simulink model "Linear_System"  (R2020a)
settings: Solver=ode4  StartTime=0.0  StopTime=10.0  RelTol=1e-3
values from neighbouring files (symbols this model uses):
  A = [0 0 0 1 0 0 ... (first row only)    [Aircraft_parameters.m]
  B = [0 0 ... (first row only)    [Aircraft_parameters.m]
  C = eye(3,6)    [Aircraft_parameters.m]
  L = place(A', C', pl)'    [main.m]
  use_output = 0    [main.m]
  use_state = 1    [main.m]
  x_bar = [0 0 0 0 0 0]'    [Aircraft_parameters.m]
  x_inital = x0-x_bar    [Aircraft_parameters.m]
undefined symbols (not defined in the file or in its folder): K
settings Model: Creator=james  LastModifiedBy=connor

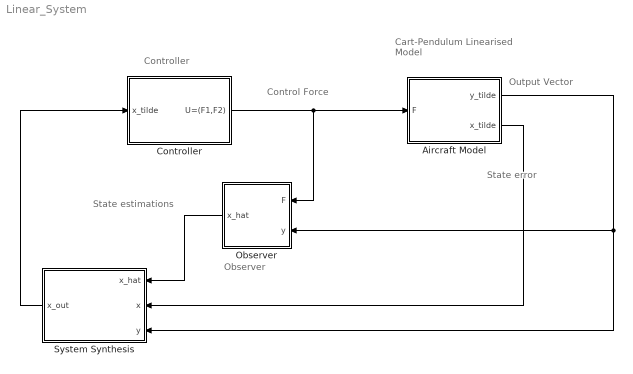
== system Linear_System ==
  note: Control Force
  note: Controller
  note: Cart-Pendulum
      | Linearised Model
  note: Output Vector
  note: Observer
  note: State error
  note: State estimations
  "Aircraft Model " : Subsystem
  Controller : Subsystem
  Observer : Subsystem
  System Synthesis : Subsystem
  wires:
  Controller/1(U=(F1,F2)) -> Observer/1(F), "Aircraft Model "/1(F)
  "Aircraft Model "/1(y_tilde) -> System Synthesis/3(y), Observer/2(y)
  "Aircraft Model "/2(x_tilde) -> System Synthesis/2(x)
  Observer/1(x_hat) -> System Synthesis/1(x_hat)
  System Synthesis/1(x_out) -> Controller/1(x_tilde)

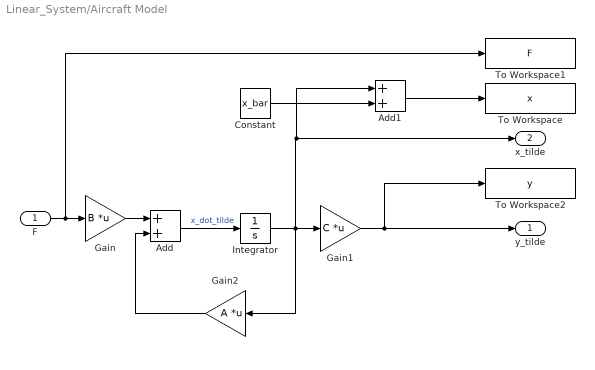
== system Linear_System/Aircraft Model  ==
  F : Inport
  Add : Sum
  Add1 : Sum
  Constant : Constant  Value=x_bar
  Gain : Gain  Gain=B  Multiplication=Matrix(K*u)
  Gain1 : Gain  Gain=C  Multiplication=Matrix(K*u)
  Gain2 : Gain  Gain=A  Multiplication=Matrix(K*u)
  Integrator : Integrator  InitialCondition=x_inital
  To Workspace : ToWorkspace  VariableName=x  SampleTime=-1
  To Workspace1 : ToWorkspace  VariableName=F  SampleTime=-1
  To Workspace2 : ToWorkspace  VariableName=y  SampleTime=-1
  y_tilde : Outport
  x_tilde : Outport  Port=2
  wires:
  F/1 -> Gain/1, To Workspace1/1
  Gain/1 -> Add/1
  Add/1 -> Integrator/1  "x_dot_tilde"
  Gain2/1 -> Add/2
  Integrator/1 -> Gain2/1, Add1/1, x_tilde/1, Gain1/1
  Gain1/1 -> y_tilde/1, To Workspace2/1
  Add1/1 -> To Workspace/1
  Constant/1 -> Add1/2

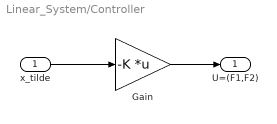
== system Linear_System/Controller ==
  x_tilde : Inport
  Gain : Gain  Gain=-K  Multiplication=Matrix(K*u)
  U=(F1,F2) : Outport
  wires:
  x_tilde/1 -> Gain/1
  Gain/1 -> U=(F1,F2)/1

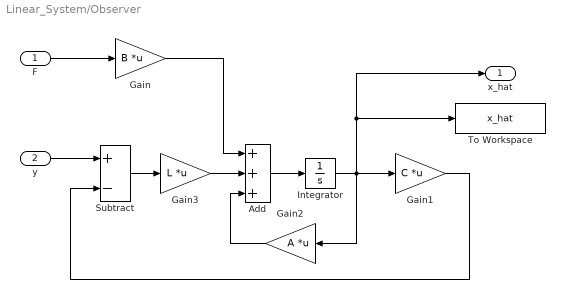
== system Linear_System/Observer ==
  F : Inport
  y : Inport  Port=2
  Add : Sum  Inputs=3
  Gain : Gain  Gain=B  Multiplication=Matrix(K*u)
  Gain1 : Gain  Gain=C  Multiplication=Matrix(K*u)
  Gain2 : Gain  Gain=A  Multiplication=Matrix(K*u)
  Gain3 : Gain  Gain=L  Multiplication=Matrix(K*u)
  Integrator : Integrator
  Subtract : Sum  Inputs=+-
  To Workspace : ToWorkspace  VariableName=x_hat  SampleTime=-1
  x_hat : Outport
  wires:
  y/1 -> Subtract/1
  F/1 -> Gain/1
  Gain/1 -> Add/1
  Gain1/1 -> Subtract/2
  Gain2/1 -> Add/3
  Add/1 -> Integrator/1
  Integrator/1 -> Gain2/1, To Workspace/1, x_hat/1, Gain1/1
  Gain3/1 -> Add/2
  Subtract/1 -> Gain3/1

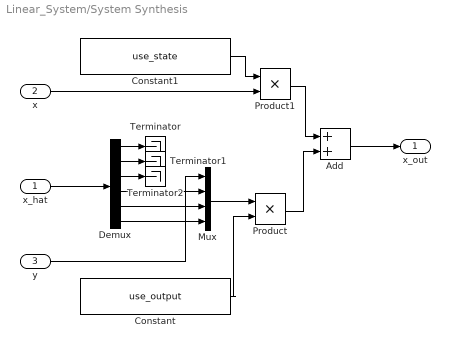
== system Linear_System/System Synthesis ==
  x_hat : Inport
  x : Inport  Port=2
  y : Inport  Port=3
  Add : Sum
  Constant : Constant  Value=use_output
  Constant1 : Constant  Value=use_state
  Demux : Demux  Outputs=6
  Mux : Mux
  Product : Product
  Product1 : Product
  Terminator : Terminator
  Terminator1 : Terminator
  Terminator2 : Terminator
  x_out : Outport
  wires:
  Demux/2 -> Terminator1/1
  Demux/1 -> Terminator/1
  x_hat/1 -> Demux/1
  y/1 -> Mux/1
  Constant/1 -> Product/2
  Mux/1 -> Product/1
  Constant1/1 -> Product1/1
  x/1 -> Product1/2
  Product1/1 -> Add/1
  Add/1 -> x_out/1
  Product/1 -> Add/2
  Demux/6 -> Mux/4
  Demux/5 -> Mux/3
  Demux/4 -> Mux/2
  Demux/3 -> Terminator2/1
